simulink model "TP2"  (R2024a)
settings: Solver=ode4  StartTime=0.0  StopTime=60  FixedStep=0.0001  RelTol=1e-3
libraries: slpidlib x8
settings Model: Creator=Lucas  LastModifiedBy=wenjun
settings DebuggingCC: UnconnectedInputMsg=warning  UnconnectedOutputMsg=warning  UnconnectedLineMsg=warning
settings ModelReferenceCC: EnableRefExpFcnMdlSchedulingChecks=on
settings RTWCC: GPUComputeCapability=3.5  DLArmComputeVersion=19.05

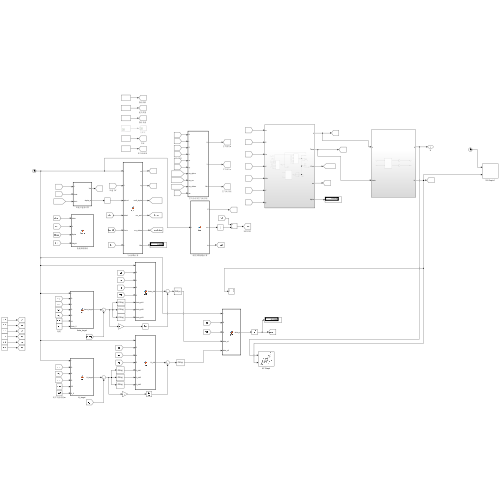
[thumbnail: Simulink's stored preview of the top-level diagram]
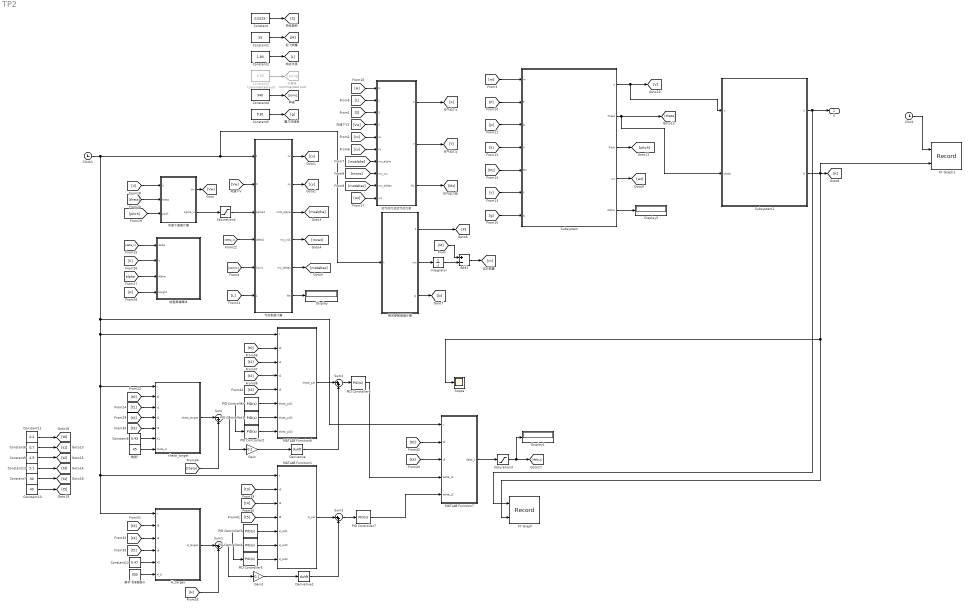
== system TP2 ==
  Add1 : Sum  Inputs=+-
  Clock : Clock
  Clock1 : Clock
  Constant : Constant  Value=0.0225
  Constant1 : Constant  Value=55
  Constant10 : Constant  Value=40
  Constant11 : Constant  Value=0.2
  Constant12 : Constant  Value=0.47
  Constant13 : Constant  Value=5.1
  Constant2 : Constant  Value=1.83
  Constant3 : Constant  Commented=on  Value=0.55
  Constant4 : Constant  Value=340
  Constant5 : Constant  Value=9.81
  Constant6 : Constant  Value=0.43
  Constant7 : Constant  Value=30
  Constant8 : Constant  Value=0.7
  Constant9 : Constant  Value=2.5
  Derivative : Derivative
  Derivative1 : Derivative
  Display : Display
  Display1 : Display
  Display3 : Display
  Gain : Gain  Gain=0.2
  Gain1 : Gain  Gain=0.1
  H_target : MATLAB Function  TreatAsAtomicUnit=on
  Integrator : Integrator
  MATLAB Function1 : MATLAB Function  TreatAsAtomicUnit=on
  MATLAB Function6 : MATLAB Function  TreatAsAtomicUnit=on
  MATLAB Function7 : MATLAB Function  TreatAsAtomicUnit=on
  PID Controller : slpidlib/PID Controller  Controller=PID  Form=Parallel  TimeDomain=Continuous-time  UseExternalTs=off  SampleTime=-1  IntegratorMethod=Forward Euler  FilterMethod=Forward Euler  ControllerParametersSource=internal  P=5  I=0  UseKiTs=off  D=1.5  UseExternalDerivativeSource=off  N=800  UseFilter=on  TunerSelectOption=Transfer Function Based (PID Tuner App)  InitialConditionSource=internal  InitialConditionForIntegrator=0  InitialConditionForFilter=0  DifferentiatorICPrevScaledInput=0  ExternalReset=none  TrackingMode=off  Kt=1  LimitOutput=off  SatLimitsSource=internal  UpperSaturationLimit=inf  LowerSaturationLimit=-inf  LinearizeAsGain=on  AntiWindupMode=none  Kb=1  LimitIntegrator=off  UpperIntegratorSaturationLimit=inf  LowerIntegratorSaturationLimit=-inf  POutMin=[]  POutMax=[]  IOutMin=[]  IOutMax=[]  DOutMin=[]  DOutMax=[]  NOutMin=[]  NOutMax=[]  SumOutMin=[]  SumOutMax=[]  SaturationOutMin=[]  SaturationOutMax=[]  PParamMin=[]  PParamMax=[]  IParamMin=[]  IParamMax=[]  DParamMin=[]  DParamMax=[]  NParamMin=[]  NParamMax=[]  KbParamMin=[]  KbParamMax=[]  KtParamMin=[]  KtParamMax=[]  KbOutMin=[]  KbOutMax=[]  KtOutMin=[]  KtOutMax=[]  IntegratorOutMin=[]  IntegratorOutMax=[]  FilterOutMin=[]  FilterOutMax=[]  SumI1OutMin=[]  SumI1OutMax=[]  SumI2OutMin=[]  SumI2OutMax=[]  SumI3OutMin=[]  SumI3OutMax=[]  SumI4OutMin=[]  SumI4OutMax=[]  SumDOutMin=[]  SumDOutMax=[]  DifferentiatorOutMin=[]  DifferentiatorOutMax=[]  FilterDiffOutCoefMin=[]  FilterDiffOutCoefMax=[]  ReciprocalOutMin=[]  ReciprocalOutMax=[]  SumDenOutMin=[]  SumDenOutMax=[]  SumNumOutMin=[]  SumNumOutMax=[]  DivideOutMin=[]  DivideOutMax=[]  UdiffTsProdOutMin=[]  UdiffTsProdOutMax=[]  NTsProdOutMin=[]  NTsProdOutMax=[]  UintegralTsProdOutMin=[]  UintegralTsProdOutMax=[]  UngainTsProdOutMin=[]  UngainTsProdOutMax=[]  ClampingZeroOutDataTypeStr=Inherit: Inherit via back propagation  ClampingZeroOutMin=[]  ClampingZeroOutMax=[]  FilterDenConstantOutDataTypeStr=Inherit: Inherit via back propagation  FilterDenConstantOutMin=[]  FilterDenConstantOutMax=[]  PCopyOutDataTypeStr=Inherit: Inherit via back propagation  PCopyOutMin=[]  PCopyOutMax=[]  NCopyOutDataTypeStr=Inherit: Inherit via back propagation  NCopyOutMin=[]  NCopyOutMax=[]  IntegratorContinuousStateAttributes=''  IntegratorStateMustResolveToSignalObject=off  IntegratorRTWStateStorageClass=Auto  FilterContinuousStateAttributes=''  FilterStateMustResolveToSignalObject=off  FilterRTWStateStorageClass=Auto  ParallelPVariant=InternalParameters  IdealPVariant=Disabled  IVariant=InternalParameters  DVariant=InternalParameters  IntegratorVariant=Continuous  SatVariant=Disabled  AWVariant=Passthrough  PCopyVariant=Disabled  TRVariant=Disabled  FdbkBlocksVariant=Forward  IdealPFdbkVariant=Disabled  SatFdbkVariant=Disabled  DerivativeFilterVariant=ContFilter  NVariant=InternalParameters  NCopyVariant=Disabled  FilterICVariant=InternalICsFilter  IntegratorICVariant=InternalICs  ExternalResetVariant=Disabled  TRSumVariant=Passthrough  SumFdbkVariant=Disabled  SumVariant=Sum_PID  TsampFilterVariant=InternalTs  TsampNgainVariant=Passthrough  TsampIntegralVariant=Disabled_SignalSpec  ExternalSaturationOutDataTypeStr=Inherit: Same as second input  DerivativeSourceVariant=ErrorSignal
  PID Controller1 : slpidlib/PID Controller  Controller=PID  Form=Parallel  TimeDomain=Continuous-time  UseExternalTs=off  SampleTime=-1  IntegratorMethod=Forward Euler  FilterMethod=Forward Euler  ControllerParametersSource=internal  P=3.5  I=1.2  UseKiTs=off  D=1.25  UseExternalDerivativeSource=off  N=800  UseFilter=on  TunerSelectOption=Transfer Function Based (PID Tuner App)  InitialConditionSource=internal  InitialConditionForIntegrator=0  InitialConditionForFilter=0  DifferentiatorICPrevScaledInput=0  ExternalReset=none  TrackingMode=off  Kt=1  LimitOutput=off  SatLimitsSource=internal  UpperSaturationLimit=inf  LowerSaturationLimit=-inf  LinearizeAsGain=on  AntiWindupMode=none  Kb=1  LimitIntegrator=off  UpperIntegratorSaturationLimit=inf  LowerIntegratorSaturationLimit=-inf  POutMin=[]  POutMax=[]  IOutMin=[]  IOutMax=[]  DOutMin=[]  DOutMax=[]  NOutMin=[]  NOutMax=[]  SumOutMin=[]  SumOutMax=[]  SaturationOutMin=[]  SaturationOutMax=[]  PParamMin=[]  PParamMax=[]  IParamMin=[]  IParamMax=[]  DParamMin=[]  DParamMax=[]  NParamMin=[]  NParamMax=[]  KbParamMin=[]  KbParamMax=[]  KtParamMin=[]  KtParamMax=[]  KbOutMin=[]  KbOutMax=[]  KtOutMin=[]  KtOutMax=[]  IntegratorOutMin=[]  IntegratorOutMax=[]  FilterOutMin=[]  FilterOutMax=[]  SumI1OutMin=[]  SumI1OutMax=[]  SumI2OutMin=[]  SumI2OutMax=[]  SumI3OutMin=[]  SumI3OutMax=[]  SumI4OutMin=[]  SumI4OutMax=[]  SumDOutMin=[]  SumDOutMax=[]  DifferentiatorOutMin=[]  DifferentiatorOutMax=[]  FilterDiffOutCoefMin=[]  FilterDiffOutCoefMax=[]  ReciprocalOutMin=[]  ReciprocalOutMax=[]  SumDenOutMin=[]  SumDenOutMax=[]  SumNumOutMin=[]  SumNumOutMax=[]  DivideOutMin=[]  DivideOutMax=[]  UdiffTsProdOutMin=[]  UdiffTsProdOutMax=[]  NTsProdOutMin=[]  NTsProdOutMax=[]  UintegralTsProdOutMin=[]  UintegralTsProdOutMax=[]  UngainTsProdOutMin=[]  UngainTsProdOutMax=[]  ClampingZeroOutDataTypeStr=Inherit: Inherit via back propagation  ClampingZeroOutMin=[]  ClampingZeroOutMax=[]  FilterDenConstantOutDataTypeStr=Inherit: Inherit via back propagation  FilterDenConstantOutMin=[]  FilterDenConstantOutMax=[]  PCopyOutDataTypeStr=Inherit: Inherit via back propagation  PCopyOutMin=[]  PCopyOutMax=[]  NCopyOutDataTypeStr=Inherit: Inherit via back propagation  NCopyOutMin=[]  NCopyOutMax=[]  IntegratorContinuousStateAttributes=''  IntegratorStateMustResolveToSignalObject=off  IntegratorRTWStateStorageClass=Auto  FilterContinuousStateAttributes=''  FilterStateMustResolveToSignalObject=off  FilterRTWStateStorageClass=Auto  ParallelPVariant=InternalParameters  IdealPVariant=Disabled  IVariant=InternalParameters  DVariant=InternalParameters  IntegratorVariant=Continuous  SatVariant=Disabled  AWVariant=Passthrough  PCopyVariant=Disabled  TRVariant=Disabled  FdbkBlocksVariant=Forward  IdealPFdbkVariant=Disabled  SatFdbkVariant=Disabled  DerivativeFilterVariant=ContFilter  NVariant=InternalParameters  NCopyVariant=Disabled  FilterICVariant=InternalICsFilter  IntegratorICVariant=InternalICs  ExternalResetVariant=Disabled  TRSumVariant=Passthrough  SumFdbkVariant=Disabled  SumVariant=Sum_PID  TsampFilterVariant=InternalTs  TsampNgainVariant=Passthrough  TsampIntegralVariant=Disabled_SignalSpec  ExternalSaturationOutDataTypeStr=Inherit: Same as second input  DerivativeSourceVariant=ErrorSignal
  PID Controller2 : slpidlib/PID Controller  Controller=PID  Form=Parallel  TimeDomain=Continuous-time  UseExternalTs=off  SampleTime=-1  IntegratorMethod=Forward Euler  FilterMethod=Forward Euler  ControllerParametersSource=internal  P=1.8  I=0.05  UseKiTs=off  D=0.75  UseExternalDerivativeSource=off  N=900  UseFilter=on  TunerSelectOption=Transfer Function Based (PID Tuner App)  InitialConditionSource=internal  InitialConditionForIntegrator=0  InitialConditionForFilter=0  DifferentiatorICPrevScaledInput=0  ExternalReset=none  TrackingMode=off  Kt=1  LimitOutput=off  SatLimitsSource=internal  UpperSaturationLimit=inf  LowerSaturationLimit=-inf  LinearizeAsGain=on  AntiWindupMode=none  Kb=1  LimitIntegrator=off  UpperIntegratorSaturationLimit=inf  LowerIntegratorSaturationLimit=-inf  POutMin=[]  POutMax=[]  IOutMin=[]  IOutMax=[]  DOutMin=[]  DOutMax=[]  NOutMin=[]  NOutMax=[]  SumOutMin=[]  SumOutMax=[]  SaturationOutMin=[]  SaturationOutMax=[]  PParamMin=[]  PParamMax=[]  IParamMin=[]  IParamMax=[]  DParamMin=[]  DParamMax=[]  NParamMin=[]  NParamMax=[]  KbParamMin=[]  KbParamMax=[]  KtParamMin=[]  KtParamMax=[]  KbOutMin=[]  KbOutMax=[]  KtOutMin=[]  KtOutMax=[]  IntegratorOutMin=[]  IntegratorOutMax=[]  FilterOutMin=[]  FilterOutMax=[]  SumI1OutMin=[]  SumI1OutMax=[]  SumI2OutMin=[]  SumI2OutMax=[]  SumI3OutMin=[]  SumI3OutMax=[]  SumI4OutMin=[]  SumI4OutMax=[]  SumDOutMin=[]  SumDOutMax=[]  DifferentiatorOutMin=[]  DifferentiatorOutMax=[]  FilterDiffOutCoefMin=[]  FilterDiffOutCoefMax=[]  ReciprocalOutMin=[]  ReciprocalOutMax=[]  SumDenOutMin=[]  SumDenOutMax=[]  SumNumOutMin=[]  SumNumOutMax=[]  DivideOutMin=[]  DivideOutMax=[]  UdiffTsProdOutMin=[]  UdiffTsProdOutMax=[]  NTsProdOutMin=[]  NTsProdOutMax=[]  UintegralTsProdOutMin=[]  UintegralTsProdOutMax=[]  UngainTsProdOutMin=[]  UngainTsProdOutMax=[]  ClampingZeroOutDataTypeStr=Inherit: Inherit via back propagation  ClampingZeroOutMin=[]  ClampingZeroOutMax=[]  FilterDenConstantOutDataTypeStr=Inherit: Inherit via back propagation  FilterDenConstantOutMin=[]  FilterDenConstantOutMax=[]  PCopyOutDataTypeStr=Inherit: Inherit via back propagation  PCopyOutMin=[]  PCopyOutMax=[]  NCopyOutDataTypeStr=Inherit: Inherit via back propagation  NCopyOutMin=[]  NCopyOutMax=[]  IntegratorContinuousStateAttributes=''  IntegratorStateMustResolveToSignalObject=off  IntegratorRTWStateStorageClass=Auto  FilterContinuousStateAttributes=''  FilterStateMustResolveToSignalObject=off  FilterRTWStateStorageClass=Auto  ParallelPVariant=InternalParameters  IdealPVariant=Disabled  IVariant=InternalParameters  DVariant=InternalParameters  IntegratorVariant=Continuous  SatVariant=Disabled  AWVariant=Passthrough  PCopyVariant=Disabled  TRVariant=Disabled  FdbkBlocksVariant=Forward  IdealPFdbkVariant=Disabled  SatFdbkVariant=Disabled  DerivativeFilterVariant=ContFilter  NVariant=InternalParameters  NCopyVariant=Disabled  FilterICVariant=InternalICsFilter  IntegratorICVariant=InternalICs  ExternalResetVariant=Disabled  TRSumVariant=Passthrough  SumFdbkVariant=Disabled  SumVariant=Sum_PID  TsampFilterVariant=InternalTs  TsampNgainVariant=Passthrough  TsampIntegralVariant=Disabled_SignalSpec  ExternalSaturationOutDataTypeStr=Inherit: Same as second input  DerivativeSourceVariant=ErrorSignal
  PID Controller3 : slpidlib/PID Controller  Controller=PID  Form=Parallel  TimeDomain=Continuous-time  UseExternalTs=off  SampleTime=-1  IntegratorMethod=Forward Euler  FilterMethod=Forward Euler  ControllerParametersSource=internal  P=1.7  I=0.005  UseKiTs=off  D=1.5  UseExternalDerivativeSource=off  N=1000  UseFilter=on  TunerSelectOption=Transfer Function Based (PID Tuner App)  InitialConditionSource=internal  InitialConditionForIntegrator=0  InitialConditionForFilter=0  DifferentiatorICPrevScaledInput=0  ExternalReset=none  TrackingMode=off  Kt=1  LimitOutput=off  SatLimitsSource=internal  UpperSaturationLimit=inf  LowerSaturationLimit=-inf  LinearizeAsGain=on  AntiWindupMode=none  Kb=1  LimitIntegrator=off  UpperIntegratorSaturationLimit=inf  LowerIntegratorSaturationLimit=-inf  POutMin=[]  POutMax=[]  IOutMin=[]  IOutMax=[]  DOutMin=[]  DOutMax=[]  NOutMin=[]  NOutMax=[]  SumOutMin=[]  SumOutMax=[]  SaturationOutMin=[]  SaturationOutMax=[]  PParamMin=[]  PParamMax=[]  IParamMin=[]  IParamMax=[]  DParamMin=[]  DParamMax=[]  NParamMin=[]  NParamMax=[]  KbParamMin=[]  KbParamMax=[]  KtParamMin=[]  KtParamMax=[]  KbOutMin=[]  KbOutMax=[]  KtOutMin=[]  KtOutMax=[]  IntegratorOutMin=[]  IntegratorOutMax=[]  FilterOutMin=[]  FilterOutMax=[]  SumI1OutMin=[]  SumI1OutMax=[]  SumI2OutMin=[]  SumI2OutMax=[]  SumI3OutMin=[]  SumI3OutMax=[]  SumI4OutMin=[]  SumI4OutMax=[]  SumDOutMin=[]  SumDOutMax=[]  DifferentiatorOutMin=[]  DifferentiatorOutMax=[]  FilterDiffOutCoefMin=[]  FilterDiffOutCoefMax=[]  ReciprocalOutMin=[]  ReciprocalOutMax=[]  SumDenOutMin=[]  SumDenOutMax=[]  SumNumOutMin=[]  SumNumOutMax=[]  DivideOutMin=[]  DivideOutMax=[]  UdiffTsProdOutMin=[]  UdiffTsProdOutMax=[]  NTsProdOutMin=[]  NTsProdOutMax=[]  UintegralTsProdOutMin=[]  UintegralTsProdOutMax=[]  UngainTsProdOutMin=[]  UngainTsProdOutMax=[]  ClampingZeroOutDataTypeStr=Inherit: Inherit via back propagation  ClampingZeroOutMin=[]  ClampingZeroOutMax=[]  FilterDenConstantOutDataTypeStr=Inherit: Inherit via back propagation  FilterDenConstantOutMin=[]  FilterDenConstantOutMax=[]  PCopyOutDataTypeStr=Inherit: Inherit via back propagation  PCopyOutMin=[]  PCopyOutMax=[]  NCopyOutDataTypeStr=Inherit: Inherit via back propagation  NCopyOutMin=[]  NCopyOutMax=[]  IntegratorContinuousStateAttributes=''  IntegratorStateMustResolveToSignalObject=off  IntegratorRTWStateStorageClass=Auto  FilterContinuousStateAttributes=''  FilterStateMustResolveToSignalObject=off  FilterRTWStateStorageClass=Auto  ParallelPVariant=InternalParameters  IdealPVariant=Disabled  IVariant=InternalParameters  DVariant=InternalParameters  IntegratorVariant=Continuous  SatVariant=Disabled  AWVariant=Passthrough  PCopyVariant=Disabled  TRVariant=Disabled  FdbkBlocksVariant=Forward  IdealPFdbkVariant=Disabled  SatFdbkVariant=Disabled  DerivativeFilterVariant=ContFilter  NVariant=InternalParameters  NCopyVariant=Disabled  FilterICVariant=InternalICsFilter  IntegratorICVariant=InternalICs  ExternalResetVariant=Disabled  TRSumVariant=Passthrough  SumFdbkVariant=Disabled  SumVariant=Sum_PID  TsampFilterVariant=InternalTs  TsampNgainVariant=Passthrough  TsampIntegralVariant=Disabled_SignalSpec  ExternalSaturationOutDataTypeStr=Inherit: Same as second input  DerivativeSourceVariant=ErrorSignal
  PID Controller4 : slpidlib/PID Controller  Controller=PID  Form=Parallel  TimeDomain=Continuous-time  UseExternalTs=off  SampleTime=-1  IntegratorMethod=Forward Euler  FilterMethod=Forward Euler  ControllerParametersSource=internal  P=2.5  I=0.02  UseKiTs=off  D=0.8  UseExternalDerivativeSource=off  N=100  UseFilter=on  TunerSelectOption=Transfer Function Based (PID Tuner App)  InitialConditionSource=internal  InitialConditionForIntegrator=0  InitialConditionForFilter=0  DifferentiatorICPrevScaledInput=0  ExternalReset=none  TrackingMode=off  Kt=1  LimitOutput=off  SatLimitsSource=internal  UpperSaturationLimit=inf  LowerSaturationLimit=-inf  LinearizeAsGain=on  AntiWindupMode=none  Kb=1  LimitIntegrator=off  UpperIntegratorSaturationLimit=inf  LowerIntegratorSaturationLimit=-inf  POutMin=[]  POutMax=[]  IOutMin=[]  IOutMax=[]  DOutMin=[]  DOutMax=[]  NOutMin=[]  NOutMax=[]  SumOutMin=[]  SumOutMax=[]  SaturationOutMin=[]  SaturationOutMax=[]  PParamMin=[]  PParamMax=[]  IParamMin=[]  IParamMax=[]  DParamMin=[]  DParamMax=[]  NParamMin=[]  NParamMax=[]  KbParamMin=[]  KbParamMax=[]  KtParamMin=[]  KtParamMax=[]  KbOutMin=[]  KbOutMax=[]  KtOutMin=[]  KtOutMax=[]  IntegratorOutMin=[]  IntegratorOutMax=[]  FilterOutMin=[]  FilterOutMax=[]  SumI1OutMin=[]  SumI1OutMax=[]  SumI2OutMin=[]  SumI2OutMax=[]  SumI3OutMin=[]  SumI3OutMax=[]  SumI4OutMin=[]  SumI4OutMax=[]  SumDOutMin=[]  SumDOutMax=[]  DifferentiatorOutMin=[]  DifferentiatorOutMax=[]  FilterDiffOutCoefMin=[]  FilterDiffOutCoefMax=[]  ReciprocalOutMin=[]  ReciprocalOutMax=[]  SumDenOutMin=[]  SumDenOutMax=[]  SumNumOutMin=[]  SumNumOutMax=[]  DivideOutMin=[]  DivideOutMax=[]  UdiffTsProdOutMin=[]  UdiffTsProdOutMax=[]  NTsProdOutMin=[]  NTsProdOutMax=[]  UintegralTsProdOutMin=[]  UintegralTsProdOutMax=[]  UngainTsProdOutMin=[]  UngainTsProdOutMax=[]  ClampingZeroOutDataTypeStr=Inherit: Inherit via back propagation  ClampingZeroOutMin=[]  ClampingZeroOutMax=[]  FilterDenConstantOutDataTypeStr=Inherit: Inherit via back propagation  FilterDenConstantOutMin=[]  FilterDenConstantOutMax=[]  PCopyOutDataTypeStr=Inherit: Inherit via back propagation  PCopyOutMin=[]  PCopyOutMax=[]  NCopyOutDataTypeStr=Inherit: Inherit via back propagation  NCopyOutMin=[]  NCopyOutMax=[]  IntegratorContinuousStateAttributes=''  IntegratorStateMustResolveToSignalObject=off  IntegratorRTWStateStorageClass=Auto  FilterContinuousStateAttributes=''  FilterStateMustResolveToSignalObject=off  FilterRTWStateStorageClass=Auto  ParallelPVariant=InternalParameters  IdealPVariant=Disabled  IVariant=InternalParameters  DVariant=InternalParameters  IntegratorVariant=Continuous  SatVariant=Disabled  AWVariant=Passthrough  PCopyVariant=Disabled  TRVariant=Disabled  FdbkBlocksVariant=Forward  IdealPFdbkVariant=Disabled  SatFdbkVariant=Disabled  DerivativeFilterVariant=ContFilter  NVariant=InternalParameters  NCopyVariant=Disabled  FilterICVariant=InternalICsFilter  IntegratorICVariant=InternalICs  ExternalResetVariant=Disabled  TRSumVariant=Passthrough  SumFdbkVariant=Disabled  SumVariant=Sum_PID  TsampFilterVariant=InternalTs  TsampNgainVariant=Passthrough  TsampIntegralVariant=Disabled_SignalSpec  ExternalSaturationOutDataTypeStr=Inherit: Same as second input  DerivativeSourceVariant=ErrorSignal
  PID Controller5 : slpidlib/PID Controller  Controller=PID  Form=Parallel  TimeDomain=Continuous-time  UseExternalTs=off  SampleTime=-1  IntegratorMethod=Forward Euler  FilterMethod=Forward Euler  ControllerParametersSource=internal  P=2  I=0.01  UseKiTs=off  D=1.2  UseExternalDerivativeSource=off  N=5000  UseFilter=on  TunerSelectOption=Transfer Function Based (PID Tuner App)  InitialConditionSource=internal  InitialConditionForIntegrator=0  InitialConditionForFilter=0  DifferentiatorICPrevScaledInput=0  ExternalReset=none  TrackingMode=off  Kt=1  LimitOutput=off  SatLimitsSource=internal  UpperSaturationLimit=inf  LowerSaturationLimit=-inf  LinearizeAsGain=on  AntiWindupMode=none  Kb=1  LimitIntegrator=off  UpperIntegratorSaturationLimit=inf  LowerIntegratorSaturationLimit=-inf  POutMin=[]  POutMax=[]  IOutMin=[]  IOutMax=[]  DOutMin=[]  DOutMax=[]  NOutMin=[]  NOutMax=[]  SumOutMin=[]  SumOutMax=[]  SaturationOutMin=[]  SaturationOutMax=[]  PParamMin=[]  PParamMax=[]  IParamMin=[]  IParamMax=[]  DParamMin=[]  DParamMax=[]  NParamMin=[]  NParamMax=[]  KbParamMin=[]  KbParamMax=[]  KtParamMin=[]  KtParamMax=[]  KbOutMin=[]  KbOutMax=[]  KtOutMin=[]  KtOutMax=[]  IntegratorOutMin=[]  IntegratorOutMax=[]  FilterOutMin=[]  FilterOutMax=[]  SumI1OutMin=[]  SumI1OutMax=[]  SumI2OutMin=[]  SumI2OutMax=[]  SumI3OutMin=[]  SumI3OutMax=[]  SumI4OutMin=[]  SumI4OutMax=[]  SumDOutMin=[]  SumDOutMax=[]  DifferentiatorOutMin=[]  DifferentiatorOutMax=[]  FilterDiffOutCoefMin=[]  FilterDiffOutCoefMax=[]  ReciprocalOutMin=[]  ReciprocalOutMax=[]  SumDenOutMin=[]  SumDenOutMax=[]  SumNumOutMin=[]  SumNumOutMax=[]  DivideOutMin=[]  DivideOutMax=[]  UdiffTsProdOutMin=[]  UdiffTsProdOutMax=[]  NTsProdOutMin=[]  NTsProdOutMax=[]  UintegralTsProdOutMin=[]  UintegralTsProdOutMax=[]  UngainTsProdOutMin=[]  UngainTsProdOutMax=[]  ClampingZeroOutDataTypeStr=Inherit: Inherit via back propagation  ClampingZeroOutMin=[]  ClampingZeroOutMax=[]  FilterDenConstantOutDataTypeStr=Inherit: Inherit via back propagation  FilterDenConstantOutMin=[]  FilterDenConstantOutMax=[]  PCopyOutDataTypeStr=Inherit: Inherit via back propagation  PCopyOutMin=[]  PCopyOutMax=[]  NCopyOutDataTypeStr=Inherit: Inherit via back propagation  NCopyOutMin=[]  NCopyOutMax=[]  IntegratorContinuousStateAttributes=''  IntegratorStateMustResolveToSignalObject=off  IntegratorRTWStateStorageClass=Auto  FilterContinuousStateAttributes=''  FilterStateMustResolveToSignalObject=off  FilterRTWStateStorageClass=Auto  ParallelPVariant=InternalParameters  IdealPVariant=Disabled  IVariant=InternalParameters  DVariant=InternalParameters  IntegratorVariant=Continuous  SatVariant=Disabled  AWVariant=Passthrough  PCopyVariant=Disabled  TRVariant=Disabled  FdbkBlocksVariant=Forward  IdealPFdbkVariant=Disabled  SatFdbkVariant=Disabled  DerivativeFilterVariant=ContFilter  NVariant=InternalParameters  NCopyVariant=Disabled  FilterICVariant=InternalICsFilter  IntegratorICVariant=InternalICs  ExternalResetVariant=Disabled  TRSumVariant=Passthrough  SumFdbkVariant=Disabled  SumVariant=Sum_PID  TsampFilterVariant=InternalTs  TsampNgainVariant=Passthrough  TsampIntegralVariant=Disabled_SignalSpec  ExternalSaturationOutDataTypeStr=Inherit: Same as second input  DerivativeSourceVariant=ErrorSignal
  PID Controller6 : slpidlib/PID Controller  Controller=PID  Form=Parallel  TimeDomain=Continuous-time  UseExternalTs=off  SampleTime=-1  IntegratorMethod=Forward Euler  FilterMethod=Forward Euler  ControllerParametersSource=internal  P=0.085  I=0  UseKiTs=off  D=0.0095  UseExternalDerivativeSource=off  N=100  UseFilter=on  TunerSelectOption=Transfer Function Based (PID Tuner App)  InitialConditionSource=internal  InitialConditionForIntegrator=0  InitialConditionForFilter=0  DifferentiatorICPrevScaledInput=0  ExternalReset=none  TrackingMode=off  Kt=1  LimitOutput=off  SatLimitsSource=internal  UpperSaturationLimit=inf  LowerSaturationLimit=-inf  LinearizeAsGain=on  AntiWindupMode=none  Kb=1  LimitIntegrator=off  UpperIntegratorSaturationLimit=inf  LowerIntegratorSaturationLimit=-inf  POutMin=[]  POutMax=[]  IOutMin=[]  IOutMax=[]  DOutMin=[]  DOutMax=[]  NOutMin=[]  NOutMax=[]  SumOutMin=[]  SumOutMax=[]  SaturationOutMin=[]  SaturationOutMax=[]  PParamMin=[]  PParamMax=[]  IParamMin=[]  IParamMax=[]  DParamMin=[]  DParamMax=[]  NParamMin=[]  NParamMax=[]  KbParamMin=[]  KbParamMax=[]  KtParamMin=[]  KtParamMax=[]  KbOutMin=[]  KbOutMax=[]  KtOutMin=[]  KtOutMax=[]  IntegratorOutMin=[]  IntegratorOutMax=[]  FilterOutMin=[]  FilterOutMax=[]  SumI1OutMin=[]  SumI1OutMax=[]  SumI2OutMin=[]  SumI2OutMax=[]  SumI3OutMin=[]  SumI3OutMax=[]  SumI4OutMin=[]  SumI4OutMax=[]  SumDOutMin=[]  SumDOutMax=[]  DifferentiatorOutMin=[]  DifferentiatorOutMax=[]  FilterDiffOutCoefMin=[]  FilterDiffOutCoefMax=[]  ReciprocalOutMin=[]  ReciprocalOutMax=[]  SumDenOutMin=[]  SumDenOutMax=[]  SumNumOutMin=[]  SumNumOutMax=[]  DivideOutMin=[]  DivideOutMax=[]  UdiffTsProdOutMin=[]  UdiffTsProdOutMax=[]  NTsProdOutMin=[]  NTsProdOutMax=[]  UintegralTsProdOutMin=[]  UintegralTsProdOutMax=[]  UngainTsProdOutMin=[]  UngainTsProdOutMax=[]  ClampingZeroOutDataTypeStr=Inherit: Inherit via back propagation  ClampingZeroOutMin=[]  ClampingZeroOutMax=[]  FilterDenConstantOutDataTypeStr=Inherit: Inherit via back propagation  FilterDenConstantOutMin=[]  FilterDenConstantOutMax=[]  PCopyOutDataTypeStr=Inherit: Inherit via back propagation  PCopyOutMin=[]  PCopyOutMax=[]  NCopyOutDataTypeStr=Inherit: Inherit via back propagation  NCopyOutMin=[]  NCopyOutMax=[]  IntegratorContinuousStateAttributes=''  IntegratorStateMustResolveToSignalObject=off  IntegratorRTWStateStorageClass=Auto  FilterContinuousStateAttributes=''  FilterStateMustResolveToSignalObject=off  FilterRTWStateStorageClass=Auto  ParallelPVariant=InternalParameters  IdealPVariant=Disabled  IVariant=InternalParameters  DVariant=InternalParameters  IntegratorVariant=Continuous  SatVariant=Disabled  AWVariant=Passthrough  PCopyVariant=Disabled  TRVariant=Disabled  FdbkBlocksVariant=Forward  IdealPFdbkVariant=Disabled  SatFdbkVariant=Disabled  DerivativeFilterVariant=ContFilter  NVariant=InternalParameters  NCopyVariant=Disabled  FilterICVariant=InternalICsFilter  IntegratorICVariant=InternalICs  ExternalResetVariant=Disabled  TRSumVariant=Passthrough  SumFdbkVariant=Disabled  SumVariant=Sum_PID  TsampFilterVariant=InternalTs  TsampNgainVariant=Passthrough  TsampIntegralVariant=Disabled_SignalSpec  ExternalSaturationOutDataTypeStr=Inherit: Same as second input  DerivativeSourceVariant=ErrorSignal
  PID Controller7 : slpidlib/PID Controller  Controller=PID  Form=Parallel  TimeDomain=Continuous-time  UseExternalTs=off  SampleTime=-1  IntegratorMethod=Forward Euler  FilterMethod=Forward Euler  ControllerParametersSource=internal  P=0.00618  I=0.00005  UseKiTs=off  D=0.0015  UseExternalDerivativeSource=off  N=1000  UseFilter=on  TunerSelectOption=Transfer Function Based (PID Tuner App)  InitialConditionSource=internal  InitialConditionForIntegrator=0  InitialConditionForFilter=0  DifferentiatorICPrevScaledInput=0  ExternalReset=none  TrackingMode=off  Kt=1  LimitOutput=off  SatLimitsSource=internal  UpperSaturationLimit=inf  LowerSaturationLimit=-inf  LinearizeAsGain=on  AntiWindupMode=none  Kb=1  LimitIntegrator=off  UpperIntegratorSaturationLimit=inf  LowerIntegratorSaturationLimit=-inf  POutMin=[]  POutMax=[]  IOutMin=[]  IOutMax=[]  DOutMin=[]  DOutMax=[]  NOutMin=[]  NOutMax=[]  SumOutMin=[]  SumOutMax=[]  SaturationOutMin=[]  SaturationOutMax=[]  PParamMin=[]  PParamMax=[]  IParamMin=[]  IParamMax=[]  DParamMin=[]  DParamMax=[]  NParamMin=[]  NParamMax=[]  KbParamMin=[]  KbParamMax=[]  KtParamMin=[]  KtParamMax=[]  KbOutMin=[]  KbOutMax=[]  KtOutMin=[]  KtOutMax=[]  IntegratorOutMin=[]  IntegratorOutMax=[]  FilterOutMin=[]  FilterOutMax=[]  SumI1OutMin=[]  SumI1OutMax=[]  SumI2OutMin=[]  SumI2OutMax=[]  SumI3OutMin=[]  SumI3OutMax=[]  SumI4OutMin=[]  SumI4OutMax=[]  SumDOutMin=[]  SumDOutMax=[]  DifferentiatorOutMin=[]  DifferentiatorOutMax=[]  FilterDiffOutCoefMin=[]  FilterDiffOutCoefMax=[]  ReciprocalOutMin=[]  ReciprocalOutMax=[]  SumDenOutMin=[]  SumDenOutMax=[]  SumNumOutMin=[]  SumNumOutMax=[]  DivideOutMin=[]  DivideOutMax=[]  UdiffTsProdOutMin=[]  UdiffTsProdOutMax=[]  NTsProdOutMin=[]  NTsProdOutMax=[]  UintegralTsProdOutMin=[]  UintegralTsProdOutMax=[]  UngainTsProdOutMin=[]  UngainTsProdOutMax=[]  ClampingZeroOutDataTypeStr=Inherit: Inherit via back propagation  ClampingZeroOutMin=[]  ClampingZeroOutMax=[]  FilterDenConstantOutDataTypeStr=Inherit: Inherit via back propagation  FilterDenConstantOutMin=[]  FilterDenConstantOutMax=[]  PCopyOutDataTypeStr=Inherit: Inherit via back propagation  PCopyOutMin=[]  PCopyOutMax=[]  NCopyOutDataTypeStr=Inherit: Inherit via back propagation  NCopyOutMin=[]  NCopyOutMax=[]  IntegratorContinuousStateAttributes=''  IntegratorStateMustResolveToSignalObject=off  IntegratorRTWStateStorageClass=Auto  FilterContinuousStateAttributes=''  FilterStateMustResolveToSignalObject=off  FilterRTWStateStorageClass=Auto  ParallelPVariant=InternalParameters  IdealPVariant=Disabled  IVariant=InternalParameters  DVariant=InternalParameters  IntegratorVariant=Continuous  SatVariant=Disabled  AWVariant=Passthrough  PCopyVariant=Disabled  TRVariant=Disabled  FdbkBlocksVariant=Forward  IdealPFdbkVariant=Disabled  SatFdbkVariant=Disabled  DerivativeFilterVariant=ContFilter  NVariant=InternalParameters  NCopyVariant=Disabled  FilterICVariant=InternalICsFilter  IntegratorICVariant=InternalICs  ExternalResetVariant=Disabled  TRSumVariant=Passthrough  SumFdbkVariant=Disabled  SumVariant=Sum_PID  TsampFilterVariant=InternalTs  TsampNgainVariant=Passthrough  TsampIntegralVariant=Disabled_SignalSpec  ExternalSaturationOutDataTypeStr=Inherit: Same as second input  DerivativeSourceVariant=ErrorSignal
  Saturation3 : Saturate  UpperLimit=9.9*pi/180  LowerLimit=-9.9*pi/180
  Saturation4 : Saturate  UpperLimit=9.9*pi/180  LowerLimit=-9.9*pi/180
  Scope : Scope
  Subsystem : Subsystem
  Subsystem1 : Subsystem
  Sum : Sum  Inputs=|-+
  Sum1 : Sum  Inputs=|-+
  Sum2 : Sum  Inputs=|++
  Sum3 : Sum  Inputs=|++
  XY Graph : Record  FileSettingsInternal="{\"entries\":[{\"content\":{\"excelSettings\":{\"content\":{},\"type\":\"Streamout.ExcelSettings\"}},\"type\":\"Streamout.FileSettingStorage\",\"uuid\":\"\"}],\"packageUris\":[\"http:\\/\\/schema.mathworks.com\\/mf0\\/streamout_blocks\\/R2020a\"],\"version\":\"1.0\"}"  Layout=[1 1]  SignalsInternal="{\"entries\":[{\"content\":{\"signals\":[{\"content\":{\"blockPath\":[],\"dimensions\":[1],\"domain\":\"\",\"lineColor\":\"#edb120\",\"plots\":[ 1 ],\"port\":1,\"sid\":[\"\"],\"signalID\":1,\"signalName\":\"Subsystem1:1\"},\"type\":\"RecordBlkView.Signal\",\"uuid\":\"\"},{\"content\":{\"blockPath\":[],\"dimensions\":[1],\"domain\":\"\",\"lineColor\":\"#7e2f8e\",\"plots\":[ 1 ],\"port\":2,\"sid\":[\"\"],\"signalID\":2,\"signalName\":\"Subsystem1:2\"},\"type\":\"RecordBlkView.Signal\",\"uuid\":\"\"}]},\"type\":\"RecordBlkView.InputSignals\",\"uuid\":\"\"}],\"packageUris\":[\"http:\\/\\/schema.mathworks.com\\/mf0\\/streamout_blocks\\/R2020a\"],\"version\":\"1.0\"}"  VisualizationBindings="{\"xyplotplugin\":{\"info\":[{\"series\":[{\"bindingParametersList\":[{\"parameter\":\"X-Axis\",\"signalID\":1,\"signalName\":\"Subsystem1:1\"},{\"parameter\":\"Y-Axis\",\"signalID\":2,\"signalName\":\"Subsystem1:2\"}],\"seriesID\":0}],\"subplotID\":1}]}}"  CompatibilityTag=XY
  XY Graph1 : Record  FileSettingsInternal="{\"entries\":[{\"content\":{\"excelSettings\":{\"content\":{},\"type\":\"Streamout.ExcelSettings\"}},\"type\":\"Streamout.FileSettingStorage\",\"uuid\":\"\"}],\"packageUris\":[\"http:\\/\\/schema.mathworks.com\\/mf0\\/streamout_blocks\\/R2020a\"],\"version\":\"1.0\"}"  Layout=[1 1]  SignalsInternal="{\"entries\":[{\"content\":{\"signals\":[{\"content\":{\"blockPath\":[],\"dimensions\":[1],\"domain\":\"\",\"lineColor\":\"#edb120\",\"plots\":[ 1 ],\"port\":1,\"sid\":[\"\"],\"signalID\":1,\"signalName\":\"Clock\"},\"type\":\"RecordBlkView.Signal\",\"uuid\":\"\"},{\"content\":{\"blockPath\":[],\"dimensions\":[1],\"domain\":\"\",\"lineColor\":\"#7e2f8e\",\"plots\":[ 1 ],\"port\":2,\"sid\":[\"\"],\"signalID\":2,\"signalName\":\"Subsystem1:2\"},\"type\":\"RecordBlkView.Signal\",\"uuid\":\"\"}]},\"type\":\"RecordBlkView.InputSignals\",\"uuid\":\"\"}],\"packageUris\":[\"http:\\/\\/schema.mathworks.com\\/mf0\\/streamout_blocks\\/R2020a\"],\"version\":\"1.0\"}"  VisualizationBindings="{\"xyplotplugin\":{\"info\":[{\"series\":[{\"bindingParametersList\":[{\"parameter\":\"X-Axis\",\"signalID\":1,\"signalName\":\"Clock\"},{\"parameter\":\"Y-Axis\",\"signalID\":2,\"signalName\":\"Subsystem1:2\"}],\"seriesID\":0}],\"subplotID\":1}]}}"  CompatibilityTag=XY
  theta_target : MATLAB Function  TreatAsAtomicUnit=on
  检查报错模块 : MATLAB Function  TreatAsAtomicUnit=on
  毛翼展 : Goto  Commented=on  GotoTag=Lwing
  气动系数计算 : MATLAB Function  TreatAsAtomicUnit=on
  相关参数插值计算 : MATLAB Function  TreatAsAtomicUnit=on
  空气动力及空气动力矩 : MATLAB Function  TreatAsAtomicUnit=on
  角度° : Constant  Value=45
  风速下速度计算 : MATLAB Function  TreatAsAtomicUnit=on
  高平飞段高度m : Constant  Value=300
  X : Outport
  wires:
  Subsystem/1(V) -> Subsystem1/1(V), [V]
  Subsystem/2(Theta) -> Subsystem1/2(theta), [theta]
  Subsystem1/1(X) -> XY Graph/1, X/1
  Constant/1 -> [S]
  [L] -> 空气动力及空气动力矩/2(L)
  Add1/1 -> [m]
  [S] -> 空气动力及空气动力矩/3(S)
  气动系数计算/5(mz_deltaz) -> [mzdeltaz]
  Integrator/1 -> Add1/2
  Clock1/1 -> H_target/1(t), MATLAB Function1/1(t), theta_target/1(t), MATLAB Function6/1(t), MATLAB Function7/1(t), 相关参数插值计算/1(t), 气动系数计算/1(t)
  空气动力及空气动力矩/1(X) -> [X]
  [M] -> Add1/1
  相关参数插值计算/2(mc) -> Integrator/1
  气动系数计算/1(cx) -> [cx]
  Constant2/1 -> [L]
  空气动力及空气动力矩/3(Mz) -> [Mz]
  [cx] -> 空气动力及空气动力矩/5(cx)
  [sonic] -> 气动系数计算/5(Sonic)
  Constant5/1 -> [g]
  气动系数计算/3(mz0_alpha) -> [mzalpha]
  Constant4/1 -> [sonic]
  [Vw] -> 气动系数计算/2(V)
  风速下速度计算/2(alpha_w) -> Saturation4/1
  空气动力及空气动力矩/2(Y) -> [Y]
  [cy] -> 空气动力及空气动力矩/6(cy)
  气动系数计算/2(cy) -> [cy]
  [mzdeltaz] -> 空气动力及空气动力矩/9(mz_deltaz)
  风速下速度计算/1(Vw) -> [Vw]
  Constant1/1 -> [M]
  [mzwz] -> 空气动力及空气动力矩/8(mz_wz)
  Constant3/1 -> 毛翼展/1
  气动系数计算/4(mz_wz1) -> [mzwz]
  [Vw] -> 空气动力及空气动力矩/4(V)
  [mzalpha] -> 空气动力及空气动力矩/7(mz_alpha)
  [m] -> Subsystem/1(m)
  相关参数插值计算/1(P) -> [P]
  [P] -> Subsystem/2(P)
  相关参数插值计算/3(Jz) -> [Jz]
  [Jz] -> Subsystem/3(Jz)
  [X] -> Subsystem/4(X)
  [Y] -> Subsystem/6(Y)
  [Mz] -> Subsystem/5(Mz)
  [g] -> Subsystem/7(g)
  Subsystem1/2(H) -> XY Graph1/2, Scope/1, XY Graph/2, [H]
  [H] -> 空气动力及空气动力矩/1(H)
  Subsystem/4(wz) -> [wz]
  [wz] -> 空气动力及空气动力矩/10(wz)
  [V] -> 风速下速度计算/1(V)
  [pitch] -> 风速下速度计算/3(pitch)
  Subsystem/3(Pitch) -> [pitch]
  [theta] -> 风速下速度计算/2(theta)
  气动系数计算/6(Ma) -> Display/1
  [L] -> 气动系数计算/6(L)
  [V] -> 检查报错模块/2(V)
  [alpha] -> 检查报错模块/3(Alpha)
  [delta_z] -> 检查报错模块/1(delta)
  [H] -> 检查报错模块/4(Height)
  [delta_z] -> 气动系数计算/4(delta1)
  Constant8/1 -> [t1]
  Constant9/1 -> [t2]
  Constant11/1 -> [t0]
  Saturation4/1 -> 气动系数计算/3(alpha1)
  Clock/1 -> XY Graph1/1
  Constant7/1 -> [t4]
  Constant10/1 -> [t5]
  Constant13/1 -> [t3]
  [t0] -> theta_target/2(t0)
  [t1] -> theta_target/3(t1)
  [t2] -> theta_target/4(t2)
  [t3] -> theta_target/5(t3)
  Constant6/1 -> theta_target/6(K1)
  角度°/1 -> theta_target/7(theta_0)
  Constant12/1 -> H_target/5(K2)
  [t5] -> H_target/4(t5)
  [t4] -> H_target/3(t4)
  [t3] -> H_target/2(t3)
  高平飞段高度m/1 -> H_target/6(H_0)
  theta_target/1(theta_target) -> Sum/1
  [theta] -> Sum/2
  H_target/1(H_target) -> Sum1/1
  [H] -> Sum1/2
  Saturation3/1 -> Display1/1, [delta_z]
  MATLAB Function7/1(delta_z) -> Saturation3/1
  [t0] -> MATLAB Function6/2(t0)
  [t1] -> MATLAB Function6/3(t1)
  [t2] -> MATLAB Function6/4(t2)
  Sum/1 -> PID Controller2/1, PID Controller/1, PID Controller1/1, Gain/1
  PID Controller/1 -> MATLAB Function6/6(theta_pid1)
  PID Controller1/1 -> MATLAB Function6/7(theta_pid2)
  PID Controller2/1 -> MATLAB Function6/8(theta_pid3)
  [t3] -> MATLAB Function1/2(t3)
  [t4] -> MATLAB Function1/3(t4)
  [t5] -> MATLAB Function1/4(t5)
  PID Controller3/1 -> MATLAB Function1/5(H_pid1)
  PID Controller4/1 -> MATLAB Function1/6(H_pid2)
  Sum1/1 -> Gain1/1, PID Controller4/1, PID Controller5/1, PID Controller3/1
  MATLAB Function1/1(H_pid) -> Sum3/1
  Sum2/1 -> PID Controller6/1
  Sum3/1 -> PID Controller7/1
  [t3] -> MATLAB Function7/3(t3)
  [t0] -> MATLAB Function7/2(t0)
  PID Controller7/1 -> MATLAB Function7/5(delta_z2)
  [t3] -> MATLAB Function6/5(t3)
  Subsystem/5(Alpha) -> Display3/1
  PID Controller5/1 -> MATLAB Function1/7(H_pid3)
  Derivative/1 -> Sum2/2
  Gain/1 -> Derivative/1
  PID Controller6/1 -> MATLAB Function7/4(delta_z1)
  MATLAB Function6/1(theta_pid) -> Sum2/1
  Derivative1/1 -> Sum3/2
  Gain1/1 -> Derivative1/1

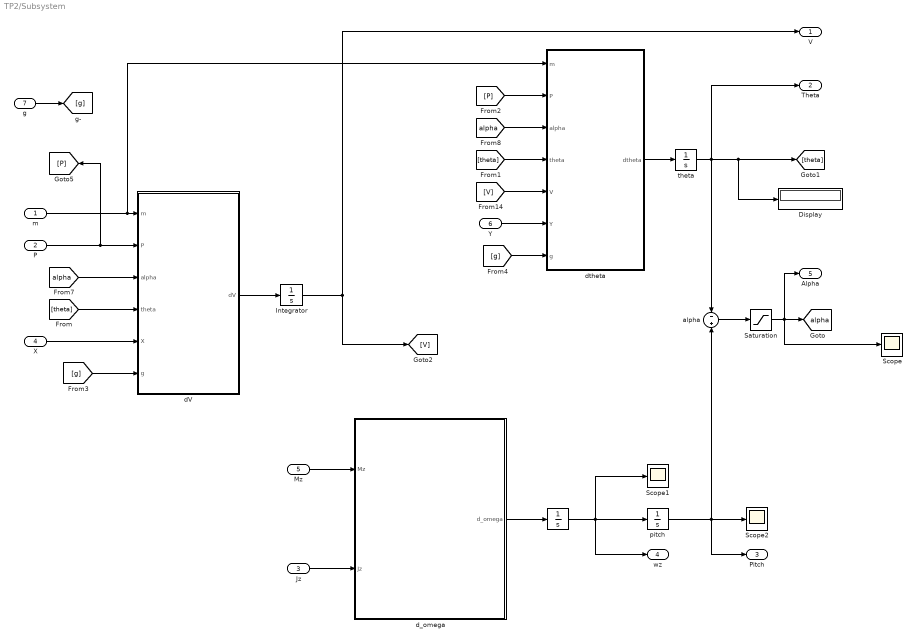
== system TP2/Subsystem ==
  m : Inport
  P : Inport  Port=2
  Jz : Inport  Port=3
  X : Inport  Port=4
  Mz : Inport  Port=5
  Y : Inport  Port=6
  g : Inport  Port=7
  " " : Integrator  UpperSaturationLimit=1  LowerSaturationLimit=-1
  Display : Display
  Integrator : Integrator  InitialCondition=20
  Saturation : Saturate  UpperLimit=10*pi/180  LowerLimit=-10*pi/180
  Scope : Scope
  Scope1 : Scope
  Scope2 : Scope
  alpha : Sum  Inputs=-+
  dV : MATLAB Function  TreatAsAtomicUnit=on
  d_omega : MATLAB Function  TreatAsAtomicUnit=on
  dtheta : MATLAB Function  TreatAsAtomicUnit=on
  pitch : Integrator  InitialCondition=45*pi/180
  theta : Integrator  InitialCondition=45*pi/180
  V : Outport
  Theta : Outport  Port=2
  Pitch : Outport  Port=3
  wz : Outport  Port=4
  Alpha : Outport  Port=5
  tag scope: alpha=global
  wires:
  d_omega/1(d_omega) -> " "/1
  Integrator/1 -> [V], V/1
  " "/1 -> wz/1, Scope1/1, pitch/1
  pitch/1 -> alpha/2, Scope2/1, Pitch/1
  m/1 -> dtheta/1(m), dV/1(m)
  [theta] -> dtheta/4(theta)
  [alpha] -> dV/3(alpha)
  dV/1(dV) -> Integrator/1
  [theta] -> dV/4(theta)
  [alpha] -> dtheta/3(alpha)
  P/1 -> dV/2(P), [P]
  alpha/1 -> Saturation/1
  dtheta/1(dtheta) -> theta/1
  Jz/1 -> d_omega/2(Jz)
  X/1 -> dV/5(X)
  [P] -> dtheta/2(P)
  [V] -> dtheta/5(V)
  Mz/1 -> d_omega/1(Mz)
  Y/1 -> dtheta/6(Y)
  g/1 -> [g]
  [g] -> dV/6(g)
  [g] -> dtheta/7(g)
  theta/1 -> alpha/1, Display/1, [theta], Theta/1
  Saturation/1 -> Alpha/1, [alpha], Scope/1

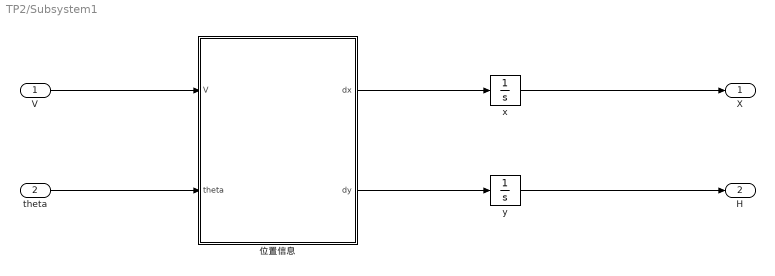
== system TP2/Subsystem1 ==
  V : Inport
  theta : Inport  Port=2
  x : Integrator
  y : Integrator  InitialCondition=2
  位置信息 : MATLAB Function  TreatAsAtomicUnit=on
  X : Outport
  H : Outport  Port=2
  wires:
  x/1 -> X/1
  y/1 -> H/1
  theta/1 -> 位置信息/2(theta)
  位置信息/1(dx) -> x/1
  位置信息/2(dy) -> y/1
  V/1 -> 位置信息/1(V)

== matlab function TP2/MATLAB Function1 ==
  data: t input; t3 input; t4 input; t5 input; H_pid1 input; H_pid2 input; H_pid output; H_pid3 input
function H_pid  = pid(t ,t3, t4, t5, H_pid1, H_pid2, H_pid3)
    H_pid = 0;
    if (t>=t3) && (t<t4)
        H_pid = H_pid1;
    elseif (t>=t4) && (t<t5)
        H_pid = H_pid2;
    elseif t>=t5
        H_pid = H_pid3;
    end

== matlab function TP2/MATLAB Function6 ==
  data: t input; t0 input; t1 input; t2 input; t3 input; theta_pid1 input; theta_pid2 input; theta_pid output; theta_pid3 input
function theta_pid  = pid(t ,t0, t1, t2, t3, theta_pid1, theta_pid2, theta_pid3)
    theta_pid = 0;
    if (t>=t0) && (t<t1)
        theta_pid=theta_pid1;
    elseif (t>=t1) && (t<t2)
        theta_pid=theta_pid2;
    elseif (t>=t2) && (t<t3)
        theta_pid=theta_pid3;
    end

== matlab function TP2/MATLAB Function7 ==
  data: t input; t0 input; t3 input; delta_z1 input; delta_z output; delta_z2 input
function delta_z  = pid(t, t0, t3, delta_z1, delta_z2)
    delta_z = 0;
    if t<t0
        delta_z =0;
    elseif (t>=t0) && (t<t3)
        delta_z=delta_z1;
    elseif t>=t3
        delta_z=delta_z2;
    end

== matlab function TP2/检查报错模块 ==
  data: delta input; V input; Alpha input; Height input
function Check(delta,V,Alpha,Height)
Mach=V/340;
if  (Mach<=0)||(Mach>=0.9)   
    error('Mach out of range');
end

% if  (Alpha<=-10*pi/180)   
%     error('Alpha too low');
% end

% if (Alpha>=10*pi/180)
%     error('Alpha too high')
% end    

if  (delta<=-10*pi/180)  
    error('Delta too low');
end

if  (delta>=10*pi/180) 
    error('Delta too high')
end    

if  (Height<=0)  
    error('Crash on the ground. Mambaout!!');
end

if  (Height>=325)
    error('Flypath too high')
end

== matlab function TP2/Subsystem/d_omega ==
  data: Mz input; d_omega output; Jz input
function d_omega = d_omega(Mz,Jz)

d_omega=Mz/Jz;

== matlab function TP2/Subsystem/dV ==
  data: m input; dV output; P input; alpha input; theta input; X input; g input
function dV = dV(m,P,alpha,theta,X,g)

dV = (P*cos(alpha)-X-m*g*sin(theta))/m;

== matlab function TP2/Subsystem/dtheta ==
  data: m input; dtheta output; P input; alpha input; theta input; V input; Y input; g input
function dtheta = dtheta(m,P,alpha,theta,V,Y,g)

dtheta = (P*sin(alpha)+Y-m*g*cos(theta))/(m*V);

== matlab function TP2/Subsystem1/位置信息 ==
  data: V input; dx output; theta input; dy output
function [dx,dy] = Kinetics(V,theta)

dx = V*cos(theta);
dy = V*sin(theta);

== matlab function TP2/H_target ==
  data: t input; t3 input; H_target output; t4 input; t5 input; K2 input; H_0 input
function H_target = fcn(t, t3, t4, t5, K2, H_0)
    H_target = H_0;
    if (t>=t3) && (t<t4)
        H_target = H_0;
    elseif (t>=t4) && (t<t5)
        H_target = (2/3)* H_0 * (exp(-K2 * (t-t4))) + (H_0/3) ;
    elseif (t>=t5)
        H_target = H_0 / 3;
    end

== matlab function TP2/theta_target ==
  data: t input; theta_target output; t0 input; t1 input; t2 input; t3 input; K1 input; theta_0 input
function theta_target = fcn(t, t0, t1, t2, t3, K1, theta_0)
    theta_start = deg2rad(theta_0);
    theta_target = theta_start;
    if (t>=t0) && (t<t1)
        theta_target = theta_start;
    elseif (t>=t1) && (t<t2)
        theta_target = theta_start * exp(- (t-t1)/K1);
    elseif (t>=t2) && (t<t3)
        theta_target = 0;
    end

== matlab function TP2/气动系数计算 ==
  data: t input; V input; alpha1 input; delta1 input; cx output; cy output; mz0_alpha output; mz_wz1 output; mz_deltaz output; Sonic input; Ma output; L input
function [cx,cy,mz0_alpha,mz_wz1,mz_deltaz,Ma] = fun(t,V,alpha1,delta1,Sonic,L)
%% 提示！输出变量"aero"是输出和，如果后面模块输入选择aero，可以在matlabfunction模块中直接写"aero.变量名"进行调用。如不需要可以直接删除
Ma=V/Sonic;
alpha=rad2deg(alpha1);
delta=rad2deg(delta1);
%% 空气动力学系数
alpha0=[0,2,4,6,8,10];%攻角 单位°
Ma0=[0.1,0.2,0.3,0.4,0.5,0.6,0.7,0.8,0.9];%Ma
if alpha <0
    flag = 1;
else
    flag= 0;
end
alpha = abs(alpha);

%% 导弹中心系数
if (t<=45)
    t_XG=[0,2.0,2.4,18.0,26.0,45.0]; 
    XG_0=[0.938,0.910,0.909,0.897,0.893,0.890]; % 单位m
    XG=interp1(t_XG,XG_0,t,'pchip');
else
    XG=0.89;
end

%% cx cy系数
cx0=[0.4298 0.4489 0.5268 0.66   0.8531 1.0911
    0.401  0.4207 0.5    0.6352 0.8307 1.0722
    0.3968 0.4167 0.4972 0.6342 0.8323 1.0773
    0.4014 0.4217 0.5033 0.6422 0.8431 1.0915
    0.4016 0.4221 0.5041 0.6438 0.8457 1.0954
    0.4101 0.4309 0.5145 0.6565 0.8619 1.1162
    0.4229 0.444  0.5384 0.6752 0.8996 1.1568
    0.4529 0.4739 0.5784 0.7121 0.9402 1.2281
    0.5546 0.5754 0.6618 0.7852 1.0764 1.3141];
cx = interp2(alpha0,Ma0,cx0,alpha,Ma,'spline');

cy0=[0 0.7268 1.5211 2.3794 3.211  4.0409
    0 0.726  1.5187 2.3752 3.2058 4.0352
    0 0.7287 1.5239 2.3826 3.2163 4.0491
    0 0.7287 1.523  2.3805 3.2133 4.0458
    0 0.733  1.5316 2.3928 3.2297 4.0667
    0 0.7427 1.5522 2.4235 3.2705 4.1192
    0 0.751  1.5697 2.4496 3.3058 4.1646
    0 0.7641 1.5977 2.4918 3.3625 4.2363
    0 0.7786 1.6424 2.5704 3.4787 4.3905];
cy = interp2(alpha0,Ma0,cy0,alpha,Ma,'spline');

if flag == 1
    cy = -cy;
end

%静稳定力矩系数
mz0_alpha0=[0   -0.0201 -0.0406 -0.0618 -0.0828 -0.1045
    0   -0.0202 -0.0407 -0.0621 -0.0831 -0.1048
    0   -0.0202 -0.0407 -0.0621 -0.083  -0.1047
    0   -0.0203 -0.041  -0.0624 -0.0833 -0.1049
    0   -0.0201 -0.0407 -0.062  -0.0825 -0.1038
    0   -0.019  -0.0384 -0.0583 -0.0776 -0.0977
    0   -0.0178 -0.0359 -0.0546 -0.0727 -0.0914
    0   -0.0171 -0.0346 -0.0529 -0.0702 -0.0885
    0   -0.0161 -0.0628 -0.0504 -0.0677 -0.0859];
mz0_alpha1=interp2(alpha0,Ma0,mz0_alpha0,alpha,Ma,'spline');

if flag ==1
    mz0_alpha1 = -mz0_alpha1;
end

mz0_alpha=mz0_alpha1+cy*(XG-0.938)/L;

%阻尼力矩导数
mz_wz_Xg938=[-0.497 -0.512 -0.528 -0.544 -0.559 -0.574
    -0.502 -0.517 -0.533 -0.549 -0.564 -0.579
    -0.506 -0.521 -0.537 -0.553 -0.568 -0.582
    -0.514 -0.529 -0.545 -0.561 -0.576 -0.591
    -0.523 -0.538 -0.554 -0.57  -0.585 -0.599
    -0.548 -0.563 -0.579 -0.594 -0.609 -0.623
    -0.578 -0.592 -0.608 -0.623 -0.638 -0.652
    -0.621 -0.635 -0.65  -0.665 -0.68  -0.694
    -0.678 -0.693 -0.709 -0.724 -0.739 -0.753];
mz_wz_Xg890=[-0.655  -0.677  -0.7  -0.722  -0.742  -0.762
    -0.662  -0.683  -0.706  -0.728  -0.749  -0.768
    -0.666  -0.688  -0.711  -0.733  -0.753  -0.773
    -0.677  -0.698  -0.721  -0.743  -0.764  -0.783
    -0.688  -0.709  -0.732  -0.754  -0.774  -0.793
    -0.718  -0.739  -0.761  -0.783  -0.803  -0.822
    -0.753  -0.774  -0.796  -0.817  -0.837  -0.855
    -0.804  -0.825  -0.846  -0.867  -0.886  -0.905
    -0.873  -0.894  -0.916  -0.938  -0.958  -0.977];
Xg_mz=[0.890,0.938];
c1 = interp2(alpha0,Ma0,mz_wz_Xg890,alpha,Ma,'spline');
c2 = interp2(alpha0,Ma0,mz_wz_Xg938,alpha,Ma,'spline');
mz_wz1=interp1(Xg_mz, [c1,c2], XG,'linear');

%操纵力矩导数
if delta<=0
    k = 1;
    delta=-delta;
else
    k = 0;
end
mz_deltaz_Xg938=[0 -0.0273 -0.0562  -0.0857  -0.1162  -0.1480
    0.0000 -0.0272  -0.0560  -0.0854  -0.1158  -0.1475
    0.0000 -0.0271  -0.0558  -0.0851  -0.1154  -0.1470
    0.0000 -0.0272  -0.0560  -0.0854  -0.1158  -0.1475
    0.0000 -0.0272  -0.0560  -0.0854  -0.1158  -0.1475
    0.0000 -0.0269  -0.0554  -0.0845  -0.1146  -0.1460
    0.0000 -0.0263  -0.0542  -0.0827  -0.1122  -0.1430
    0.0000 -0.0260  -0.0536  -0.0818  -0.1110  -0.1415
    0.0000 -0.0256  -0.0528  -0.0806  -0.1094  -0.1395];
mz_deltaz_Xg890=[0  -0.0289 -0.0595 -0.0906 -0.1228 -0.1562
    0  -0.0288 -0.0593 -0.0903 -0.1224 -0.1557
    0  -0.0287 -0.0591 -0.0900 -0.1219 -0.1551
    0  -0.0288 -0.0593 -0.0903 -0.1224 -0.1557
    0  -0.0288 -0.0593 -0.0903 -0.1224 -0.1557
    0  -0.0285 -0.0586 -0.0893 -0.1211 -0.1541
    0  -0.0279 -0.0574 -0.0874 -0.1186 -0.1509
    0  -0.0276 -0.0567 -0.0865 -0.1173 -0.1493
    0  -0.0271 -0.0559 -0.0852 -0.1156 -0.1472];
Xg_deltaz=[0.890,0.938];
c3 = interp2(alpha0,Ma0,mz_deltaz_Xg890,delta,Ma,'spline');
c4 = interp2(alpha0,Ma0,mz_deltaz_Xg938,delta,Ma,'spline');
mz_deltaz=interp1(Xg_deltaz, [c3,c4], XG,'linear');
if k==1
    mz_deltaz = -mz_deltaz;
end

== matlab function TP2/相关参数插值计算 ==
  data: t input; P output; mc output; Jz output
function [P,mc,Jz] = fun(t)


%% 推力系数
if (t<= 2.1)
    t_P1=[0,0.15,0.49,2.1];%时间
    P0_1=[3400,6320,5200,6260];%推力 单位
    P = interp1(t_P1,P0_1,t,"makima");
elseif (t>=2.1) && (t<=45)
    t_P2=[2.1,2.27,3.53,8.78,25.2,45,45.1];
    P0_2=[6260,500,450,430,420,420,0];
    P = interp1(t_P2,P0_2,t,"linear");
else
    P=0;
end

%% 发动机质量秒流量
if (t<= 45)
    t_mc=[0,2.1,2.2,45,45.1];%时间
    mc0=[2.39,2.39,0.22,0.22,0];%发动机质量秒流量 单位kg/s
    mc= interp1(t_mc,mc0,t,'pchip');
else
    mc=0;
end

%% 转动惯量系数
if (t<= 45)
    t_Jz=[0,2,2.4,10.4,18.4,22.4,30.4,34.0,45.0];%转动惯量时间
    Jz0=[8.69,8.20,8.17,8.09,8.04,8.02,8.01,8.0,8.0];% 转动惯量 单位kgms
    Jz = interp1(t_Jz,Jz0,t,'pchip');
else
    Jz=8.0;
end

== matlab function TP2/空气动力及空气动力矩 ==
  data: H input; L input; S input; X output; V input; cx input; cy input; mz_alpha input; mz_wz input; Y output; Mz output; mz_deltaz input; wz input
function [X,Y,Mz] = fcn(H,L,S,V,cx,cy,mz_alpha,mz_wz,mz_deltaz,wz)

rou=1.225*exp(-H/10700);

X=cx*0.5*rou*(V^2)*S;
Y=cy*0.5*rou*(V^2)*S;
Mz_alpha=mz_alpha*0.5*rou*(V^2)*S*L;
Mz_wz=mz_wz*wz*L*0.5*rou*(V^2)*S*L/V;
Mz_deltaz=mz_deltaz*0.5*rou*(V^2)*S*L;
Mz=Mz_alpha+Mz_wz+Mz_deltaz;

== matlab function TP2/风速下速度计算 ==
  settings: updateMethod=DISCRETE
  data: V input; Vw output; theta input; pitch input; alpha_w output
function [Vw,alpha_w] = fcn(V,theta,pitch)
Wcx=0;   % 常值风速，可以改
Wcy=0;

deltaWx0 = 0;   % 随机风速均值（m/s）
deltaWy0 = 0;

delta_deltaWx = (0.1*Wcx-0.1)/0.6744; % 风速标准差（m/s）
deltaWx = deltaWx0 + delta_deltaWx * randn();

delta_deltaWy = (0.1*Wcy-0.1)/0.6744; % 风速标准差（m/s）
deltaWy = deltaWy0 + delta_deltaWy * randn();

Wx=Wcx+deltaWx;
Wy=Wcy+deltaWy;

Vx=V*cos(theta);
Vy=V*sin(theta);

Vw=sqrt((Vx-Wx)^2+(Vy-Wy)^2);
theta_w=atan((Vy-Wy)/(Vx-Wx));
alpha_w=pitch-theta_w;
